simulink model "class_4_simulink"  (R2023b)
settings: Solver=VariableStepAuto  StartTime=0.0  StopTime=10.0  RelTol=1e-3
values from neighbouring files (symbols this model uses):
  denp = [3 1]    [class_4.m]
  h = 6.5    [class_4.m]
  nump = 2    [class_4.m]
libraries: cstblocks x3
settings Model: Creator=klysm  LastModifiedBy=klysm

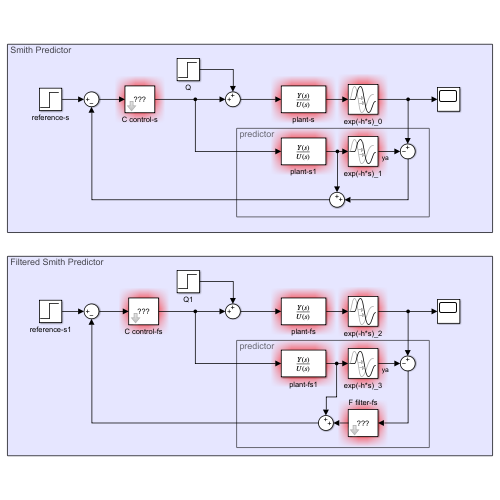
[thumbnail: Simulink's stored preview of the top-level diagram]
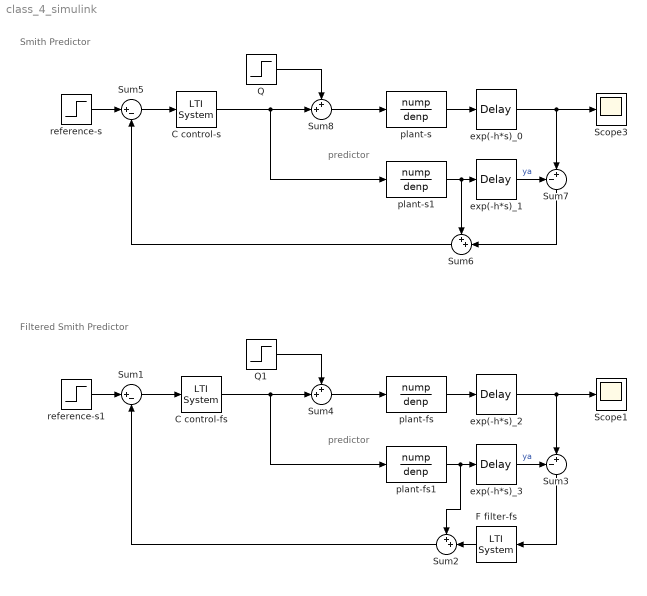
== system class_4_simulink ==
  note: Filtered Smith Predictor
  note: predictor
  note: Smith Predictor
  note: predictor
  C control-fs : cstblocks/LTI System  sys=C  IC=[]  PadeOrder=0
  C control-s : cstblocks/LTI System  sys=C  IC=[]  PadeOrder=0
  F filter-fs : cstblocks/LTI System  sys=C  IC=[]  PadeOrder=0
  Q : Step  SampleTime=0
  Q1 : Step  SampleTime=0
  Scope1 : Scope
  Scope3 : Scope
  Sum1 : Sum  Inputs=|+-
  Sum{2,4,6,8} (4 alike) : Sum  Inputs=++|
  Sum3 : Sum  Inputs=-+|
  Sum5 : Sum  Inputs=|+-
  Sum7 : Sum  Inputs=-+|
  exp(-h*s)_{0..3} (4 alike) : TransportDelay  DelayTime=h
  plant-fs : TransferFcn  Numerator=nump  Denominator=denp
  plant-fs1 : TransferFcn  Numerator=nump  Denominator=denp
  plant-s : TransferFcn  Numerator=nump  Denominator=denp
  plant-s1 : TransferFcn  Numerator=nump  Denominator=denp
  reference-s : Step  SampleTime=0
  reference-s1 : Step  SampleTime=0
  wires:
  Sum3/1 -> F filter-fs/1
  reference-s1/1 -> Sum1/1
  plant-fs1/1 -> exp(-h*s)_3/1, Sum2/1
  plant-fs/1 -> exp(-h*s)_2/1
  C control-fs/1 -> Sum4/2, plant-fs1/1
  Sum2/1 -> Sum1/2
  exp(-h*s)_3/1 -> Sum3/1  "ya"
  Sum4/1 -> plant-fs/1
  exp(-h*s)_2/1 -> Scope1/1, Sum3/2
  Sum1/1 -> C control-fs/1
  Q1/1 -> Sum4/1
  F filter-fs/1 -> Sum2/2
  Sum7/1 -> Sum6/2
  reference-s/1 -> Sum5/1
  plant-s1/1 -> Sum6/1, exp(-h*s)_1/1
  plant-s/1 -> exp(-h*s)_0/1
  Sum6/1 -> Sum5/2
  exp(-h*s)_1/1 -> Sum7/1  "ya"
  Sum8/1 -> plant-s/1
  exp(-h*s)_0/1 -> Scope3/1, Sum7/2
  Sum5/1 -> C control-s/1
  Q/1 -> Sum8/1
  C control-s/1 -> Sum8/2, plant-s1/1
